simulink model "sim_cam_1"  (R2023b)
settings: Solver=VariableStepAuto  StartTime=0.0  StopTime=Tend_slk  RelTol=1e-3
values from neighbouring files (symbols this model uses):
  param = [Ixx;Iyy;Izz;l;k;b;m]    [main_cam.m]
  Ts_slk = 0.01    [main_cam.m]
undefined symbols (not defined in the file or in its folder): ctrl_gains, x_des
libraries: px4Sensorslib x3, robotcorelib x2, uavutilslib x1
settings Model: Creator=asus  LastModifiedBy=Camilla
settings OptimizationCC: ReuseModelBlockBuffer=off

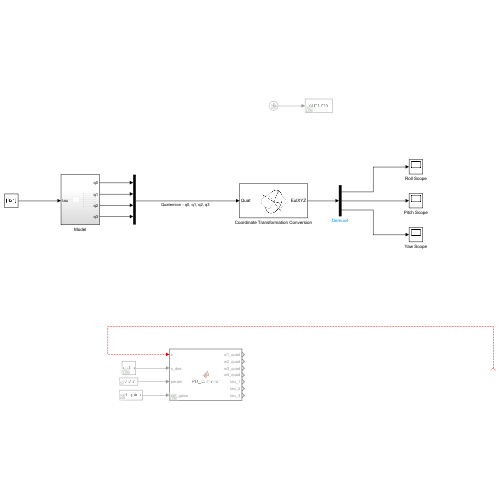
[thumbnail: Simulink's stored preview of the top-level diagram]
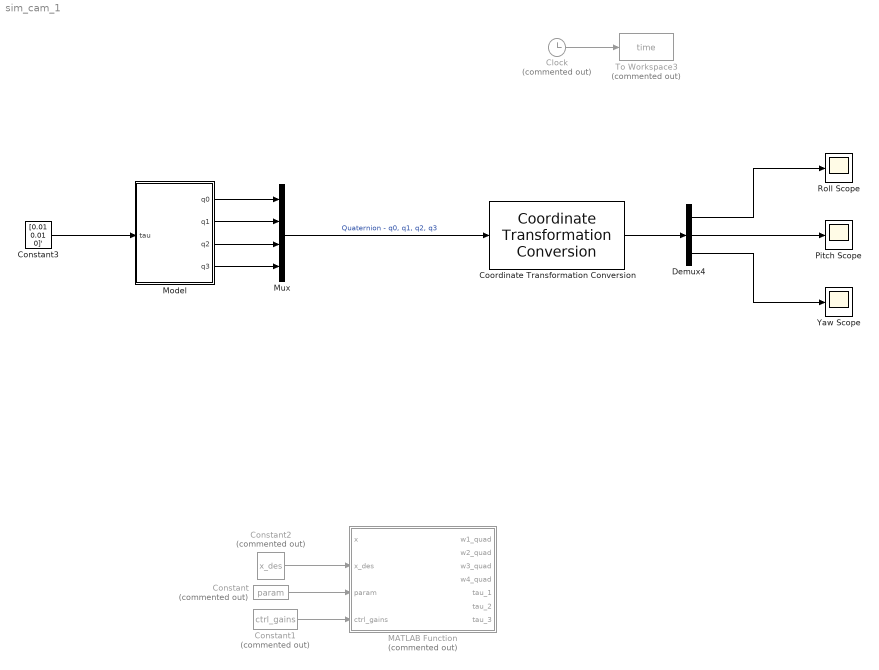
== system sim_cam_1 ==
  Clock : Clock  Commented=on
  Constant : Constant  Commented=on  Value=param
  Constant1 : Constant  Commented=on  Value=ctrl_gains
  Constant2 : Constant  Commented=on  Value=x_des
  Constant3 : Constant  Value=[0.01 0.01 0]'  VectorParams1D=off
  Coordinate Transformation Conversion : robotcorelib/Coordinate Transformation Conversion  InputRepresentation=Quaternion  InputEulerSequence=ZYX  ShowTrVecInputPort=on  OutputRepresentation=Euler Angles  OutputEulerSequence=XYZ  ShowTrVecOutputPort=on  SimulateUsing=Interpreted execution
      settings: LibrarySourceBlock=uavutilslib/Coordinate Transformation Conversion
  Demux4 : Demux  Outputs=3
  MATLAB Function : MATLAB Function  Commented=on  TreatAsAtomicUnit=on
  Model : Subsystem
  Mux : Mux
  Pitch Scope : Scope
  Roll Scope : Scope
  To Workspace3 : ToWorkspace  Commented=on  VariableName=time  SampleTime=Ts_slk
      settings: Save2DSignal=2-D array (concatenate along first dimension)
  Yaw Scope : Scope
  wires:
  Clock/1 -> To Workspace3/1
  ? -> MATLAB Function/1(x)
  Constant/1 -> MATLAB Function/3(param)
  Constant2/1 -> MATLAB Function/2(x_des)
  Constant1/1 -> MATLAB Function/4(ctrl_gains)
  Constant3/1 -> Model/1("tau ")
  Coordinate Transformation Conversion/1 -> Demux4/1
  Demux4/3 -> Yaw Scope/1
  Demux4/1 -> Roll Scope/1
  Demux4/2 -> Pitch Scope/1
  Mux/1 -> Coordinate Transformation Conversion/1  "Quaternion - q0, q1, q2, q3"
  Model/1(q0) -> Mux/1
  Model/2(q1) -> Mux/2
  Model/3(q2) -> Mux/3
  Model/4(q3) -> Mux/4

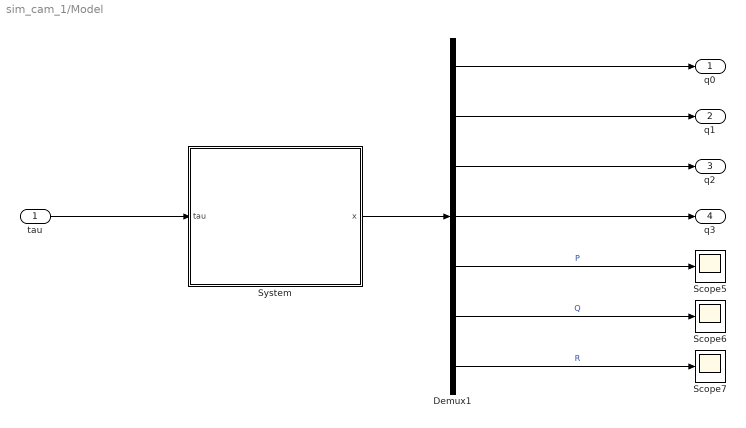
== system sim_cam_1/Model ==
  "tau " : Inport
  Demux1 : Demux  Outputs=7
  Scope5 : Scope
  Scope6 : Scope
  Scope7 : Scope
  System : Subsystem
  q0 : Outport
  q1 : Outport  Port=2
  q2 : Outport  Port=3
  q3 : Outport  Port=4
  wires:
  Demux1/5 -> Scope5/1  "P"
  Demux1/7 -> Scope7/1  "R"
  System/1(x) -> Demux1/1
  Demux1/1 -> q0/1
  "tau "/1 -> System/1("tau ")
  Demux1/6 -> Scope6/1  "Q"
  Demux1/2 -> q1/1
  Demux1/3 -> q2/1
  Demux1/4 -> q3/1

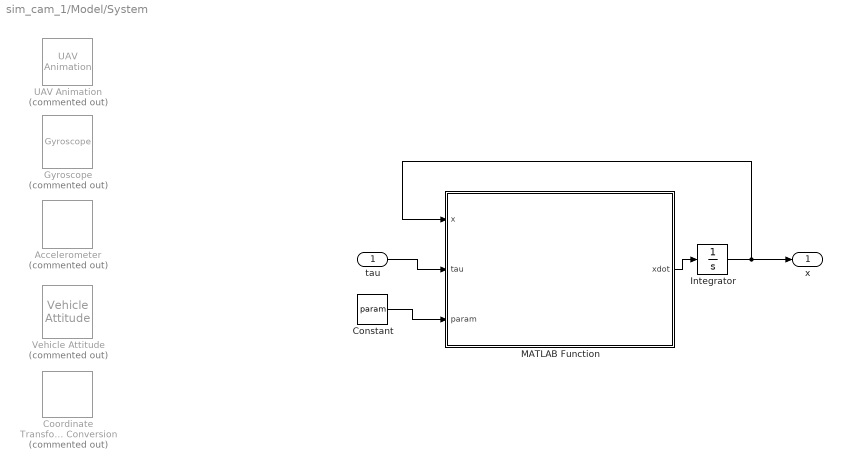
== system sim_cam_1/Model/System ==
  "tau " : Inport
  Accelerometer : px4Sensorslib/Accelerometer  Commented=on  uorbTimeStamp=off  BlockingMode=off  BlockTimeout=1e-3  sampleTime=1/250
  Constant : Constant  Value=param
  Coordinate Transformation Conversion : robotcorelib/Coordinate Transformation Conversion  Commented=on  InputRepresentation=Quaternion  InputEulerSequence=ZYX  ShowTrVecInputPort=on  OutputRepresentation=Euler Angles  OutputEulerSequence=XYZ  ShowTrVecOutputPort=on  SimulateUsing=Interpreted execution
      settings: LibrarySourceBlock=uavutilslib/Coordinate Transformation Conversion
  Gyroscope : px4Sensorslib/Gyroscope  Commented=on  uorbTimeStamp=off  BlockingMode=off  BlockTimeout=1e-3  sampleTime=1/250
  Integrator : Integrator  InitialCondition=[1 0 0 0 0 0 0]'
  MATLAB Function : MATLAB Function  TreatAsAtomicUnit=on
  UAV Animation : uavutilslib/UAV Animation  Commented=on  UAVType=Multirotor  UAVSize=1  InertialZDirection=Up  SampleTime=-1
  Vehicle Attitude : px4Sensorslib/Vehicle Attitude  Commented=on  rollRate=off  pitchRate=off  yawRate=off  quaternion=on  uorbTimeStamp=off  BlockingMode=off  BlockTimeout=0.001  sampleTime=1/250
  x : Outport
  wires:
  Integrator/1 -> x/1, MATLAB Function/1(x)
  MATLAB Function/1(xdot) -> Integrator/1
  Constant/1 -> MATLAB Function/3(param)
  "tau "/1 -> MATLAB Function/2(tau)

== matlab function sim_cam_1/Model/System/MATLAB Function ==
  data: x input; tau input; xdot output; param input
function xdot = model_cam(x, tau, param)

% This is the model inserted in the simulink, 
% I'm uploading it in a separate file too for quick reading

% Inputs:   x: state vector
%           tau: torque vector
%           param: moment of inertia
% 
% Outputs:  xdot  (derivative of the state w.r.t. time)

%% Input Data

% Parameters
g        =       9.81;           %  gravity acceleration (m/s^2)
Ixx      =       param(1,1);     %  moment of inertia 
Iyy      =       param(2,1);     %  moment of inertia
Izz      =       param(3,1);     %  moment of inertia

% States
q0       =       x(1,1);     
q1       =       x(2,1);     
q2       =       x(3,1);       
q3       =       x(4,1);     
P        =       x(5,1);     
Q        =       x(6,1);     
R        =       x(7,1);

% torques
tau_1    =       tau(1,1);   %  roll torque 
tau_2    =       tau(2,1);   %  pitch torque 
tau_3    =       tau(3,1);   %  yaw torque

%% Define useful matrices

Quaternion_Multiplication       =      [0    -P    -Q    -R; 
                                        P     0    -R     Q; 
                                        Q     R     0    -P; 
                                        R    -Q     P     0];

Quaternion      =      [q0 q1 q2 q3]';

%% Model Equations

xdot     =       zeros(7,1);

xdot(1:4,1)     =     (-1/2)*Quaternion_Multiplication*Quaternion;
xdot(5:7,1)     =     [(Iyy-Izz)*Q*R/Ixx; (Izz-Ixx)*P*R/Iyy; (Ixx-Iyy)*P*Q/Izz] + [tau_1/Ixx; tau_2/Iyy; tau_3/Izz];

== matlab function sim_cam_1/MATLAB Function ==
  data: x input; w1_quad output; x_des input; param input; w2_quad output; ctrl_gains input; w3_quad output; w4_quad output; tau_1 output; tau_2 output; tau_3 output
function [w1_quad,w2_quad,w3_quad,w4_quad, tau_1, tau_2,tau_3] = PD_controller(x,x_des,param,ctrl_gains)
% Inputs:
%           x       (model state)
%           x_des   (desired state)           
%           param   (model parameters)
%           ctrl_gains (control gains)
%
% Outputs:  
%           wi_quad     (square of i-th propeller angular velocity)


% Parameters
g        =       9.81;           %  gravity acceleration (m/s^2)
Ixx      =       param(1,1);     %  moment of inertia 
Iyy      =       param(2,1);     %  moment of inertia
Izz      =       param(3,1);     %  moment of inertia
l        =       param(4,1);     %  //TODO da stimare   
k        =       param(5,1);     %  //TODO da stimare
b        =       param(6,1);     %  //TODO da stimare
m        =       param(7,1);     %  mass (kg)

% States
phi      =       x(1,1);     %  roll angle (rad)
theta    =       x(2,1);     %  pitch angle (rad)
psi      =       x(3,1);     %  yaw angle (rad)  
phi_dot  =       x(4,1);     %  roll rate (rad/s)
theta_dot=       x(5,1);     %  pitch rate (rad/s)
psi_dot  =       x(6,1);     %  yaw rate (rad/s)  

% Target states
phi_des      =       x_des(1,1);     %  target roll angle (rad)
theta_des    =       x_des(2,1);     %  target pitch angle (rad)
psi_des      =       x_des(3,1);     %  target yaw angle (rad)  
phi_dot_des  =       x_des(4,1);     %  target roll rate (rad/s)
theta_dot_des=       x_des(5,1);     %  target pitch rate (rad/s)
psi_dot_des  =       x_des(6,1);     %  target yaw rate (rad/s) 

% Control gains
K_ph_d      =       ctrl_gains(1,1);
K_th_d      =       ctrl_gains(2,1);
K_ps_d      =       ctrl_gains(3,1);
K_ph_p      =       ctrl_gains(4,1);
K_th_p      =       ctrl_gains(5,1);
K_ps_p      =       ctrl_gains(6,1);

% Control
tau_1       =       Ixx*(K_ph_d*(phi_dot_des-phi_dot)+K_ph_p*(phi_des-phi));
tau_2       =       Iyy*(K_th_d*(theta_dot_des-theta_dot)+K_th_p*(theta_des-theta));
tau_3       =       Izz*(K_ps_d*(psi_dot_des-psi_dot)+K_ps_p*(psi_des-psi));

cph         =       cos(phi);
cth         =       cos(theta);
T           =       m*g/cth/cph;

w1_quad     =       T/(4*k)-tau_2/(2*k*l)-tau_3/(4*b);        % w1^2
w2_quad     =       T/(4*k)-tau_1/(2*k*l)+tau_3/(4*b);
w3_quad     =       T/(4*k)+tau_2/(2*k*l)-tau_3/(4*b);
w4_quad     =       T/(4*k)+tau_1/(2*k*l)+tau_3/(4*b);
